simulink model "ES8_sim"  (R2024a)
settings: Solver=VariableStepAuto  StartTime=0.0  StopTime=10.0  RelTol=1e-3
values from neighbouring files (symbols this model uses):
  A = [0 2;-4.5 -10]    [E8.m]
  B = [1 1]'    [E8.m]
  C = [1 1]    [E8.m]
  G = eye(2)    [E8.m]
  Rv = 0.01    [E8.m]
  Rw = [0 0; 0 0.01]    [E8.m]
undefined symbols (not defined in the file or in its folder): L
settings Model: Creator=stefa  LastModifiedBy=stefa

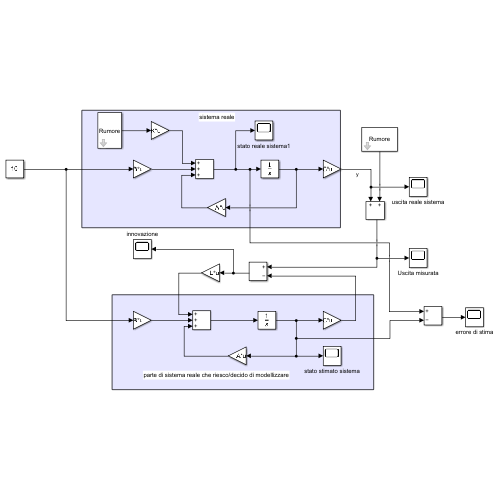
[thumbnail: Simulink's stored preview of the top-level diagram]
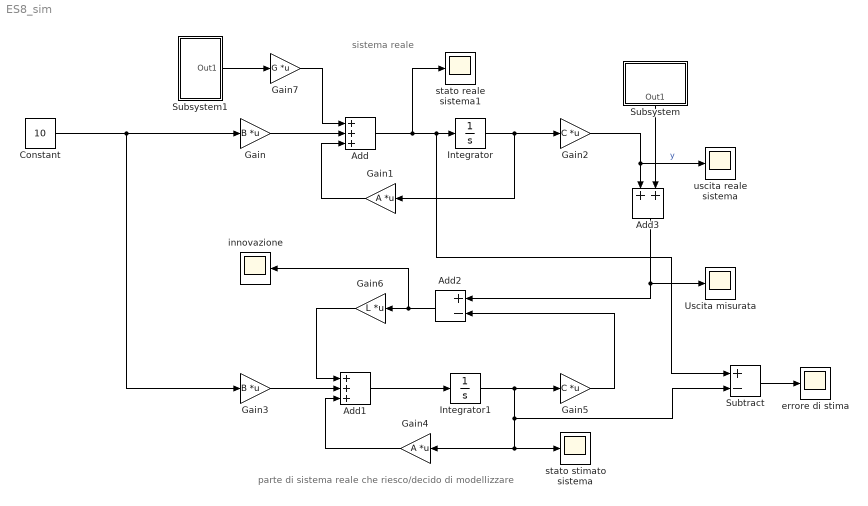
== system ES8_sim ==
  note: parte di sistema reale che riesco/decido di modellizzare
  note: sistema reale
  Add : Sum  Inputs=+++
  Add1 : Sum  Inputs=+++
  Add2 : Sum  Inputs=+-
  Add3 : Sum
  Constant : Constant  Value=10
  Gain : Gain  Gain=B  Multiplication=Matrix(K*u)
  Gain1 : Gain  Gain=A  Multiplication=Matrix(K*u)
  Gain2 : Gain  Gain=C  Multiplication=Matrix(K*u)
  Gain3 : Gain  Gain=B  Multiplication=Matrix(K*u)
  Gain4 : Gain  Gain=A  Multiplication=Matrix(K*u)
  Gain5 : Gain  Gain=C  Multiplication=Matrix(K*u)
  Gain6 : Gain  Gain=L  Multiplication=Matrix(K*u)
  Gain7 : Gain  Gain=G  Multiplication=Matrix(K*u)
  Integrator : Integrator
  Integrator1 : Integrator
  Subsystem : Subsystem  mask{mat_cov=Rv}
      mask prompts: mat_cov "Covariance Matrix"
      mask Display: disp('Rumore')
  Subsystem1 : Subsystem  mask{mat_cov=Rw}
      mask prompts: mat_cov "Covariance Matrix"
      mask Display: disp('Rumore')
  Subtract : Sum  Inputs=+-
  Uscita misurata : Scope
  errore di stima : Scope
  innovazione : Scope
  stato reale sistema1 : Scope
  stato stimato sistema : Scope
  uscita reale sistema : Scope
  wires:
  Gain/1 -> Add/2
  Add/1 -> stato reale sistema1/1, Subtract/1, Integrator/1
  Constant/1 -> Gain/1, Gain3/1
  Gain1/1 -> Add/3
  Integrator/1 -> Gain1/1, Gain2/1
  Integrator1/1 -> Subtract/2, Gain4/1, stato stimato sistema/1, Gain5/1
  Gain4/1 -> Add1/3
  Add1/1 -> Integrator1/1
  Gain3/1 -> Add1/2
  Gain6/1 -> Add1/1
  Add2/1 -> innovazione/1, Gain6/1
  Gain5/1 -> Add2/2
  Add3/1 -> Uscita misurata/1, Add2/1
  Subsystem/1(Out1) -> Add3/2
  Gain2/1 -> uscita reale sistema/1, Add3/1  "y"
  Subsystem1/1(Out1) -> Gain7/1
  Gain7/1 -> Add/1
  Subtract/1 -> errore di stima/1

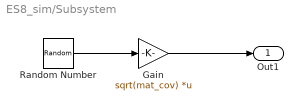
== system ES8_sim/Subsystem ==
  Gain : Gain  Gain=sqrt(mat_cov)  Multiplication=Matrix(K*u)
  Random Number : RandomNumber  Mean=zeros(size(mat_cov,1),1)  Variance=ones(size(mat_cov,1),1)  Seed=floor([1:size(mat_cov,1)].*(abs(randn(1,size(mat_cov,1))*10)+1))  SampleTime=0.001
  Out1 : Outport  VectorParamsAs1DForOutWhenUnconnected=off
  wires:
  Random Number/1 -> Gain/1
  Gain/1 -> Out1/1

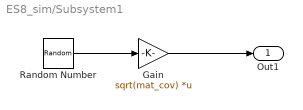
== system ES8_sim/Subsystem1 ==
  Gain : Gain  Gain=sqrt(mat_cov)  Multiplication=Matrix(K*u)
  Random Number : RandomNumber  Mean=zeros(size(mat_cov,1),1)  Variance=ones(size(mat_cov,1),1)  Seed=floor([1:size(mat_cov,1)].*(abs(randn(1,size(mat_cov,1))*10)+1))  SampleTime=0.001
  Out1 : Outport  VectorParamsAs1DForOutWhenUnconnected=off
  wires:
  Random Number/1 -> Gain/1
  Gain/1 -> Out1/1
